simulink model "robot_soccer_sim"  (R2013a)
settings: Solver=ode45  StartTime=0.0  StopTime=1000000  RelTol=1e-3
InitFcn:
  | param
undefined symbols (not defined in the file or in its folder): controller_away, controller_home, drawEnvironment_est, lowlevelctrl, P, robot_change_frames, vision_system
settings Model: Creator=beard  LastModifiedBy=beard

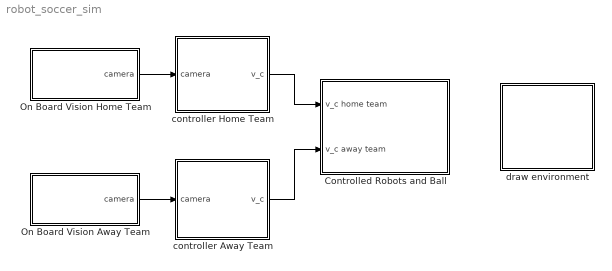
== system robot_soccer_sim ==
  "Controlled Robots and Ball " : Subsystem
      mask Display: image(imread('cmu_2002_diffbot.jpg'))
  On Board Vision Away Team : Subsystem
      mask Display: image(imread('softkinect.png'))
  On Board Vision Home Team : Subsystem
      mask Display: image(imread('softkinect.png'))
  controller Away Team : Subsystem
      mask Display: image(imread('minnowboard.png'))
  controller Home Team : Subsystem
      mask Display: image(imread('minnowboard.png'))
  draw environment : Subsystem
      mask Display: image(imread('ssl_game.jpg'))
  wires:
  controller Away Team/1(v_c) -> "Controlled Robots and Ball "/2(v_c away team)
  controller Home Team/1(v_c) -> "Controlled Robots and Ball "/1(v_c home team)
  On Board Vision Home Team/1(camera) -> controller Home Team/1(camera)
  On Board Vision Away Team/1(camera) -> controller Away Team/1(camera)

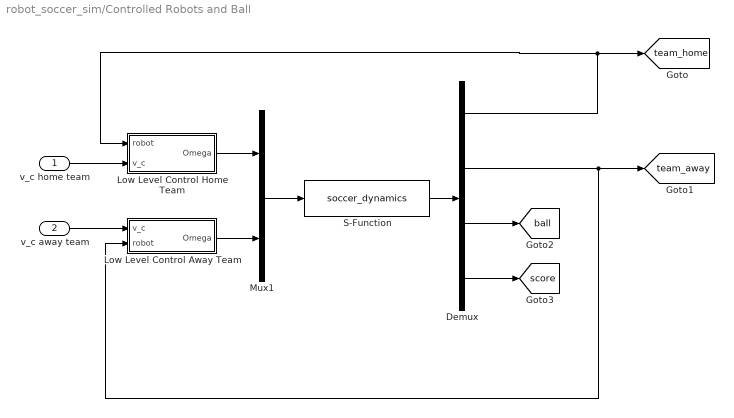
== system robot_soccer_sim/Controlled Robots and Ball  ==
  v_c home team : Inport
  v_c away team : Inport  Port=2
  Demux : Demux  Outputs=[3*P.num_robots; 3*P.num_robots; 2; 2]
  Low Level Control Home Team : Subsystem
  Low Level Control Away Team : Subsystem
  Mux1 : Mux  Inputs=2
  S-Function : S-Function  FunctionName=soccer_dynamics  Parameters=P  EnableBusSupport=off
  tag scope: ball=global, score=global, team_away=global, team_home=global
  wires:
  Demux/4 -> [score]
  v_c away team/1 -> Low Level Control Away Team/1(v_c)
  v_c home team/1 -> Low Level Control Home Team/2(v_c)
  Demux/2 -> [team_away], Low Level Control Away Team/2(robot)
  Low Level Control Away Team/1(Omega) -> Mux1/2
  Low Level Control Home Team/1(Omega) -> Mux1/1
  Demux/1 -> [team_home], Low Level Control Home Team/1(robot)
  S-Function/1 -> Demux/1
  Demux/3 -> [ball]
  Mux1/1 -> S-Function/1

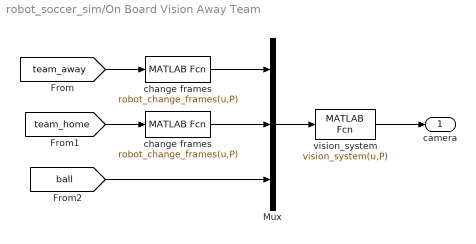
== system robot_soccer_sim/On Board Vision Away Team ==
  Mux : Mux  Inputs=3
  "change frames " : MATLABFcn  MATLABFcn=robot_change_frames(u,P)  OutputDimensions=3*P.num_robots  SampleTime=P.control_sample_rate
  "change frames " : MATLABFcn  MATLABFcn=robot_change_frames(u,P)  OutputDimensions=3*P.num_robots  SampleTime=P.control_sample_rate
  vision_system : MATLABFcn  MATLABFcn=vision_system(u,P)  OutputDimensions=(2+4*P.num_robots+2*P.num_markers)*P.num_robots  SampleTime=.01
  camera : Outport
  wires:
  Mux/1 -> vision_system/1
  vision_system/1 -> camera/1
  [team_away] -> "change frames "/1
  "change frames "/1 -> Mux/1
  [team_home] -> "change frames "/1
  "change frames "/1 -> Mux/2
  [ball] -> Mux/3

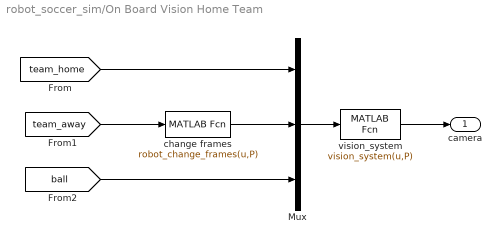
== system robot_soccer_sim/On Board Vision Home Team ==
  Mux : Mux  Inputs=3
  "change frames " : MATLABFcn  MATLABFcn=robot_change_frames(u,P)  OutputDimensions=3*P.num_robots  SampleTime=P.control_sample_rate
  vision_system : MATLABFcn  MATLABFcn=vision_system(u,P)  OutputDimensions=(2+4*P.num_robots+2*P.num_markers)*P.num_robots  SampleTime=.01
  camera : Outport
  wires:
  Mux/1 -> vision_system/1
  [team_home] -> Mux/1
  [ball] -> Mux/3
  vision_system/1 -> camera/1
  [team_away] -> "change frames "/1
  "change frames "/1 -> Mux/2

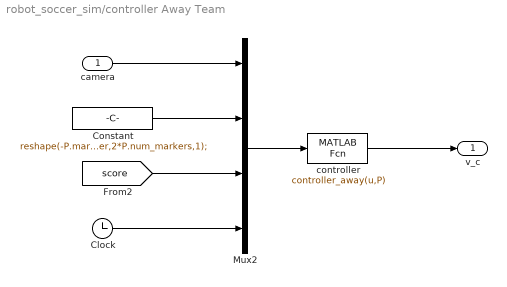
== system robot_soccer_sim/controller Away Team ==
  camera : Inport
  Clock : Clock
  Constant : Constant  Value=reshape(-P.marker,2*P.num_markers,1);
  Mux2 : Mux
  controller : MATLABFcn  MATLABFcn=controller_away(u,P)  OutputDimensions=3*P.num_robots  SampleTime=P.control_sample_rate
  v_c : Outport
  wires:
  Clock/1 -> Mux2/4
  camera/1 -> Mux2/1
  Mux2/1 -> controller/1
  controller/1 -> v_c/1
  Constant/1 -> Mux2/2
  [score] -> Mux2/3

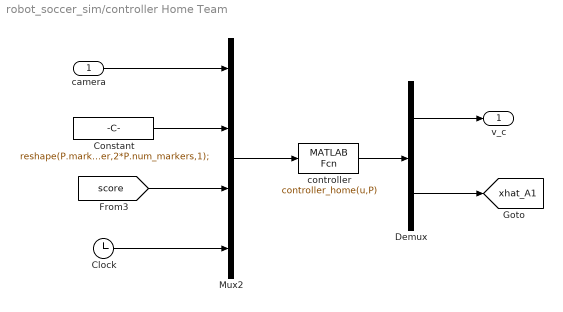
== system robot_soccer_sim/controller Home Team ==
  camera : Inport
  Clock : Clock
  Constant : Constant  Value=reshape(P.marker,2*P.num_markers,1);
  Demux : Demux  Outputs=[3*P.num_robots; 6];
  Mux2 : Mux
  controller : MATLABFcn  MATLABFcn=controller_home(u,P)  OutputDimensions="3*P.num_robots  + 6"  SampleTime=P.control_sample_rate
  v_c : Outport
  tag scope: xhat_A1=global
  wires:
  Clock/1 -> Mux2/4
  camera/1 -> Mux2/1
  Mux2/1 -> controller/1
  controller/1 -> Demux/1
  Demux/1 -> v_c/1
  Demux/2 -> [xhat_A1]
  Constant/1 -> Mux2/2
  [score] -> Mux2/3

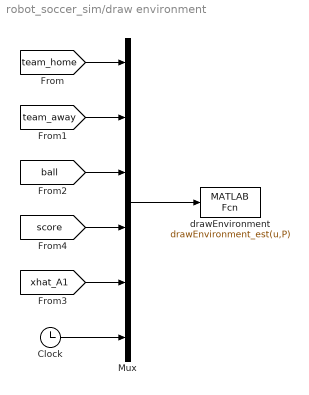
== system robot_soccer_sim/draw environment ==
  Clock : Clock
  Mux : Mux  Inputs=6
  drawEnvironment : MATLABFcn  MATLABFcn=drawEnvironment_est(u,P)  OutputDimensions=0  SampleTime=P.display_rate
  wires:
  Mux/1 -> drawEnvironment/1
  Clock/1 -> Mux/6
  [team_home] -> Mux/1
  [team_away] -> Mux/2
  [ball] -> Mux/3
  [xhat_A1] -> Mux/5
  [score] -> Mux/4

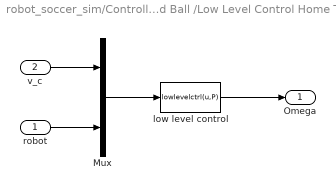
== system robot_soccer_sim/Controlled Robots and Ball /Low Level Control Home Team ==
  robot : Inport
  v_c : Inport  Port=2
  Mux : Mux  Inputs=2
  low level control : MATLABFcn  MATLABFcn=lowlevelctrl(u,P)  OutputDimensions=3*P.num_robots  SampleTime=0.01
  Omega : Outport
  wires:
  low level control/1 -> Omega/1
  Mux/1 -> low level control/1
  robot/1 -> Mux/2
  v_c/1 -> Mux/1

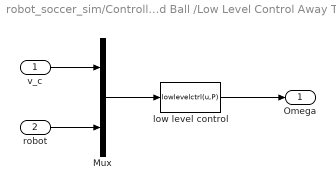
== system robot_soccer_sim/Controlled Robots and Ball /Low Level Control Away Team ==
  v_c : Inport
  robot : Inport  Port=2
  Mux : Mux  Inputs=2
  low level control : MATLABFcn  MATLABFcn=lowlevelctrl(u,P)  OutputDimensions=3*P.num_robots  SampleTime=0.01
  Omega : Outport
  wires:
  low level control/1 -> Omega/1
  Mux/1 -> low level control/1
  robot/1 -> Mux/2
  v_c/1 -> Mux/1
